simulink model "LQG_dis_red"  (R2023b)
settings: Solver=VariableStepAuto  StartTime=0.0  StopTime=200  RelTol=1e-3
undefined symbols (not defined in the file): A_red, Ad, B_total_red, Bd_u, C_ss_red, Cd, CI_red, D_ss, DI_red, DiscIntNeverNeededParam, Discrete, dVdt, K_red, Kint_red, Rn_red, sigma, step_temp, steptime, Time, Ts, Tsp_red, Ufeedforward_red, V0, Vb0, Vmax, Vmin, wd
libraries: ctrlSharedLib x1, simulink x1
settings Model: Creator=Maialen  LastModifiedBy=Maialen

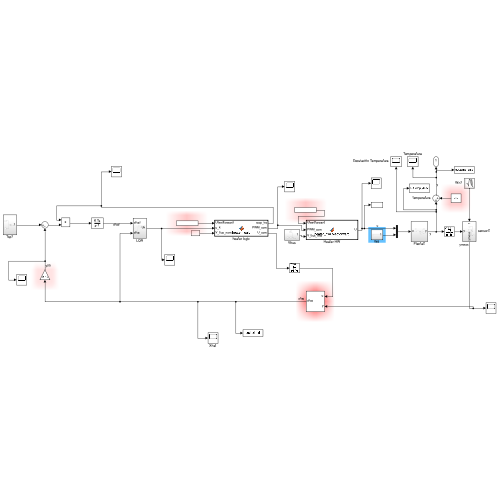
[thumbnail: Simulink's stored preview of the top-level diagram]
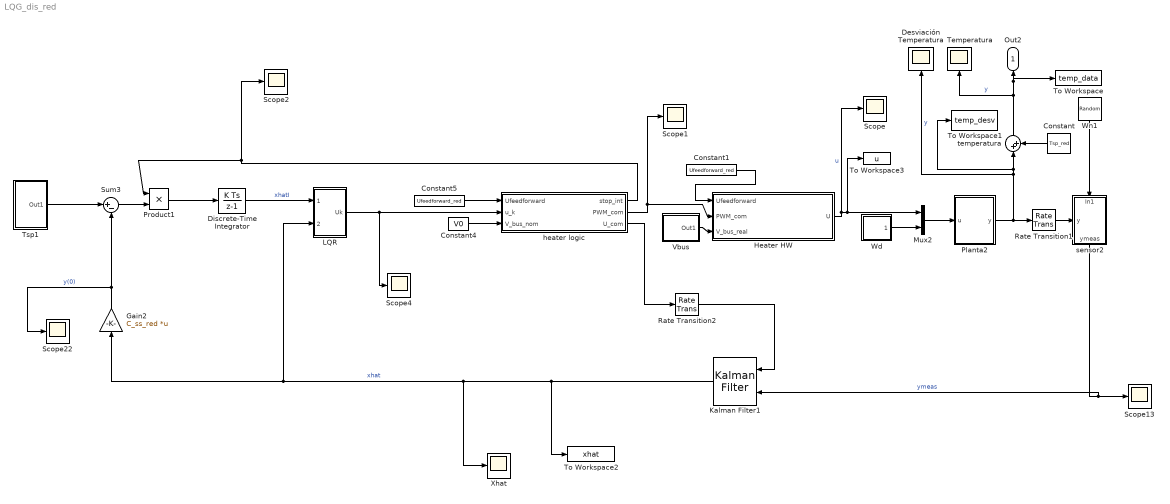
== system LQG_dis_red ==
  Constant : Constant  Value=Tsp_red  SampleTime=0
  Constant1 : Constant  Value=Ufeedforward_red  SampleTime=0
  Constant4 : Constant  Value=V0  SampleTime=0
  Constant5 : Constant  Value=Ufeedforward_red  SampleTime=0
  Desviación Temperatura : Scope
  Discrete-Time Integrator : DiscreteIntegrator  SampleTime=Ts  ICPrevOutput=DiscIntNeverNeededParam  ICPrevScaledInput=DiscIntNeverNeededParam
  Gain2 : Gain  Gain=C_ss_red  Multiplication=Matrix(K*u)
  Heater HW : MATLAB Function  TreatAsAtomicUnit=on
  Kalman Filter1 : ctrlSharedLib/Kalman Filter  TimeDomain=Discrete-Time  UseCurrentEstimator=on  ModelSource=LTI State-Space Variable  ModelSourceVariable=syskf_red  A=Ad  B=Bd_u  C=Cd  D=D_ss  NumberOfStates=1  NumberOfInputs=1  NumberOfOutputs=1  InitialEstimateSource=Dialog  X0=0  P0=10  UseK=off  UseGH=off  NumberOfProcessNoiseInputs=1  G=1  TimeInvariantG=on  H=0  TimeInvariantH=on  Q=Qn_red  TimeInvariantQ=on  R=Rn_red  TimeInvariantR=on  N=0  TimeInvariantN=on  AddInputPort=on  AddEnablePort=off  OutputEstimatedY=off  OutputP=off  Ts=1
  LQR : Subsystem
  Mux2 : Mux  Inputs=2
  Planta2 : Subsystem
  Product1 : Product
  Rate Transition1 : RateTransition  OutPortSampleTime=Ts
  Rate Transition2 : RateTransition  OutPortSampleTime=Ts
  Scope{,1..2,4,13,22} (6 alike) : Scope
  Sum3 : Sum  Inputs=|+-
  Temperatura : Scope
  To Workspace : ToWorkspace  VariableName=temp_data  SaveFormat=Timeseries  SampleTime=-1
  To Workspace1 : ToWorkspace  VariableName=temp_desv  SaveFormat=Timeseries  SampleTime=-1
  To Workspace2 : ToWorkspace  VariableName=xhat  SaveFormat=Timeseries  SampleTime=-1
  To Workspace3 : ToWorkspace  VariableName=u  SaveFormat=Timeseries  SampleTime=-1
  Tsp1 : Subsystem
  Vbus : Subsystem
  Wd : Subsystem
  Wn1 : RandomNumber  Variance=sigma^2  SampleTime=Ts
  Xhat : Scope
  heater logic : MATLAB Function  TreatAsAtomicUnit=on
  sensor2 : Subsystem
      settings: PortSchema="{\"entries\":[{\"content\":{\"sides\":[{\"content\":{\"connectorIds\":[\"In1\"]},\"type\":\"ConnectorPlacement.EquallySpacedRectSide\",\"uuid\":\"87c57665-5a3a-4a29-be31-fc3b8356ea98\"},{\"content\":{\"connectorIds\":[\"Out1\"],\"side\":\"RIGHT\"},\"type\":\"ConnectorPlacement.EquallySpacedRectSide\",\"uuid\":\"3fe956b0-7f9e-4b46-bcb6-e49be4c7e683\"},{\"content\":{\"connectorIds\":[\"In2\"],\"side\":\"TOP\"},\"type\":\"ConnectorPlacement.EquallySpacedRectSide\",\"uuid\":\"3d207620-bc84-4c0d-9751-3dea453ac424\"}]},\"type\":\"ConnectorPlacement.EquallySpacedConnector\",\"uuid\":\"7e1a59fd-e04d-40d6-8549-9ebaaabea5d7\"}],\"packageUris\":[\"http://schema.mathworks.com/mf0/Connector/R2020b\"],\"version\":\"1.0\"}"
  temperatura : Sum  Inputs=|++
  Out2 : Outport
  wires:
  Heater HW/1(U) -> Scope/1, Mux2/1, To Workspace3/1  "u"
  heater logic/3(U_com) -> Rate Transition2/1
  Constant/1 -> temperatura/2
  temperatura/1 -> To Workspace/1, Out2/1, Temperatura/1  "y"
  Planta2/1(y) -> Desviación Temperatura/1, temperatura/1, To Workspace1/1, Rate Transition1/1  "y"
  Constant1/1 -> Heater HW/1(Ufeedforward)
  Tsp1/1(Out1) -> Sum3/1
  Constant5/1 -> heater logic/1(Ufeedforward)
  Discrete-Time Integrator/1 -> LQR/1(xhatI)  "xhatI"
  LQR/1(Uk) -> Scope4/1, heater logic/2(u_k)
  Mux2/1 -> Planta2/1(u)
  Vbus/1(Out1) -> Heater HW/3(V_bus_real)
  Constant4/1 -> heater logic/3(V_bus_nom)
  Kalman Filter1/1 -> To Workspace2/1, Xhat/1, LQR/2(xhat), Gain2/1  "xhat"
  Wn1/1 -> sensor2/1(In1)
  sensor2/1(ymeas) -> Kalman Filter1/2, Scope13/1  "ymeas"
  Sum3/1 -> Product1/2
  Product1/1 -> Discrete-Time Integrator/1
  heater logic/2(PWM_com) -> Scope1/1, Heater HW/2(PWM_com)
  Gain2/1 -> Sum3/2, Scope22/1  "y(0)"
  Wd/1(Out1) -> Mux2/2
  heater logic/1(stop_int) -> Scope2/1, Product1/1
  Rate Transition1/1 -> sensor2/2(y)
  Rate Transition2/1 -> Kalman Filter1/1

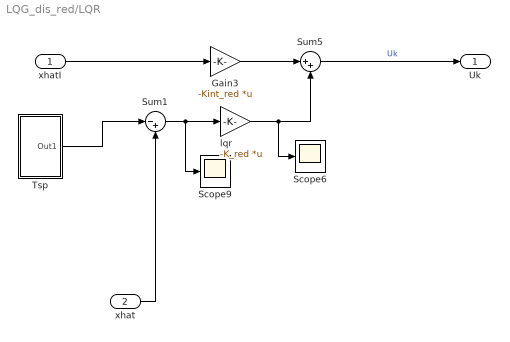
== system LQG_dis_red/LQR ==
  xhatI : Inport
  xhat : Inport  Port=2
  Gain3 : Gain  Gain=-Kint_red  Multiplication=Matrix(K*u)
  Scope6 : Scope
  Scope9 : Scope
  Sum1 : Sum  Inputs=|-+
  Sum5 : Sum  Inputs=|++
  Tsp : Subsystem
  lqr : Gain  Gain=-K_red  Multiplication=Matrix(K*u)
  Uk : Outport
  wires:
  xhatI/1 -> Gain3/1
  lqr/1 -> Scope6/1, Sum5/2
  Gain3/1 -> Sum5/1
  Sum1/1 -> Scope9/1, lqr/1
  xhat/1 -> Sum1/2
  Tsp/1(Out1) -> Sum1/1
  Sum5/1 -> Uk/1  "Uk"

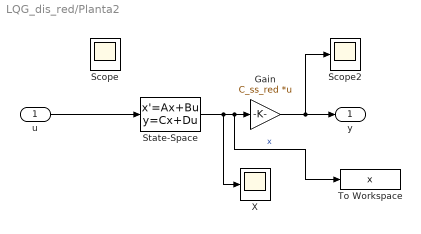
== system LQG_dis_red/Planta2 ==
  u : Inport
  Gain : Gain  Gain=C_ss_red  Multiplication=Matrix(K*u)
  Scope : Scope
  Scope2 : Scope
  State-Space : StateSpace  A=A_red  B=B_total_red  C=CI_red  D=DI_red  InitialCondition=0
  To Workspace : ToWorkspace  VariableName=x  SaveFormat=Timeseries  SampleTime=-1
  X : Scope
  y : Outport
  wires:
  Gain/1 -> Scope2/1, y/1
  State-Space/1 -> X/1, To Workspace/1, Gain/1  "x"
  u/1 -> State-Space/1

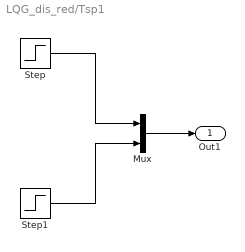
== system LQG_dis_red/Tsp1 ==
  Mux : Mux  Inputs=2
  Step : Step  Time=steptime  After=step_temp  SampleTime=0
  Step1 : Step  Time=steptime  After=step_temp  SampleTime=0
  Out1 : Outport
  wires:
  Mux/1 -> Out1/1
  Step/1 -> Mux/1
  Step1/1 -> Mux/2

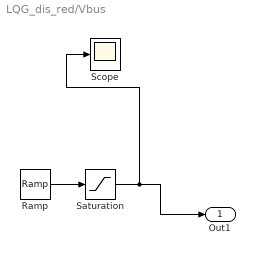
== system LQG_dis_red/Vbus ==
  Ramp : simulink/Sources/Ramp  slope=dVdt  start=steptime  InitialOutput=Vb0
  Saturation : Saturate  UpperLimit=Vmax  LowerLimit=Vmin
  Scope : Scope
  Out1 : Outport
  wires:
  Ramp/1 -> Saturation/1
  Saturation/1 -> Scope/1, Out1/1

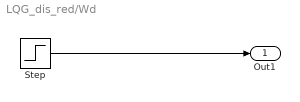
== system LQG_dis_red/Wd ==
  Step : Step  Time=steptime  After=wd  SampleTime=0
  Out1 : Outport
  wires:
  Step/1 -> Out1/1

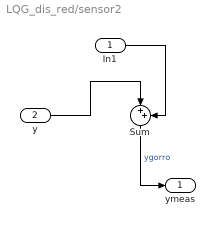
== system LQG_dis_red/sensor2 ==
  In1 : Inport
  y : Inport  Port=2
  Sum : Sum  Inputs=|++
  ymeas : Outport
  wires:
  In1/1 -> Sum/2
  y/1 -> Sum/1
  Sum/1 -> ymeas/1  "ygorro"

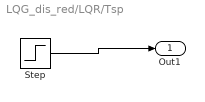
== system LQG_dis_red/LQR/Tsp ==
  Step : Step  Time=steptime  After=step_temp  SampleTime=0
  Out1 : Outport
  wires:
  Step/1 -> Out1/1

== matlab function LQG_dis_red/Heater HW ==
  data: Ufeedforward input; PWM_com input; U output; V_bus_real input
function U   = heater_hwUfeedforward( Ufeedforward, PWM_com, V_bus_real)
    R_real = [156.8; 156.8];
    
    % Potencia real entregada a la planta
    P_max_real = (V_bus_real^2) ./ R_real;

    U= PWM_com .* P_max_real - Ufeedforward;
end

== matlab function LQG_dis_red/heater logic ==
  data: stop_int output; Ufeedforward input; u_k input; PWM_com output; V_bus_nom input; U_com output
function [stop_int, PWM_com, U_com] = heater_logic(Ufeedforward, u_k, V_bus_nom)
    R0 = [ 156.8; 156.8];
    
    % Potencia máxima disponible
    P_max = (V_bus_nom^2) ./ R0;
    
    % Potencia absoluta demandada = feedforward + corrección LQR (desviación)
    P_demanda = Ufeedforward + u_k;
    
    % Saturación física
    P_limitada = max(0, min(P_max, P_demanda));
    
    % PWM lineal
    PWM_com = P_limitada ./ P_max;
    
    % Anti-windup: congela integrador si satura
    sat_arriba = P_demanda >= P_max;
    sat_abajo  = P_demanda <= 0;
    stop_int   = double(~(sat_arriba | sat_abajo));
    
    % Potencia comandada (para el Kalman)
    U_com = P_limitada - Ufeedforward;
end
